simulink model "model_vec"  (R2022b)
settings: Solver=ode4  StartTime=0.0  StopTime=1.3  FixedStep=10e-6  RelTol=1e-3
InitFcn:
  | model_
values from neighbouring files (symbols this model uses):
  f = 50    [model_.m]
  i1dn = psi2n/Lm    [model_.m]
  i1qn = sqrt(Inmax^2-i1dn^2)    [model_.m]
  J = 0.4    [model_.m]
  L1 = L1sigma+Lm    (= 0.08477)    [model_.m]
  L1sigma = 2.27e-3    (= 0.00227)    [model_.m]
  L2 = L2sigma+Lm    (= 0.08477)    [model_.m]
  L2sigma = 2.27e-3    (= 0.00227)    [model_.m]
  Lm = 82.5e-3    (= 0.0825)    [model_.m]
  pp = 2    [model_.m]
  psi2n = sqrt(psi2nre^2+psi2nim^2)    [model_.m]
  R1 = 370e-3    (= 0.37)    [model_.m]
  R2 = 225e-3    (= 0.225)    [model_.m]
  R2_vec_model = 225e-3    (= 0.225)    [model_.m]
  sigma = 1-Lm^(2)/(L1*L2)    (= 0.0528396032209)    [model_.m]
  svmFrequency = 10000    [model_.m]
  Us = 400    [model_.m]
libraries: eeTransforms x16, spsMeanLib x7, slpidlib x4, simulink x2, dspsigops x2
(part 1 of 3)
settings Model: Creator=petrzakopal  LastModifiedBy=petrzakopal

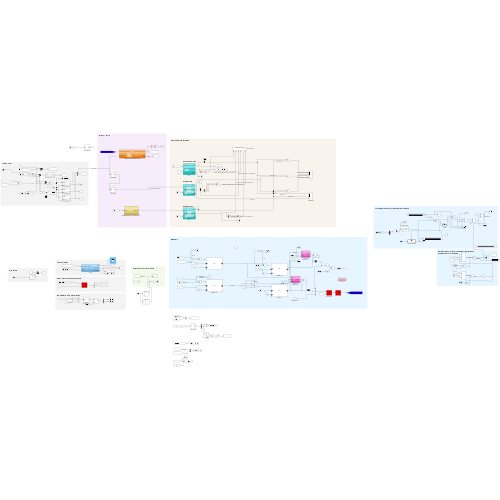
[thumbnail: Simulink's stored preview of the top-level diagram]
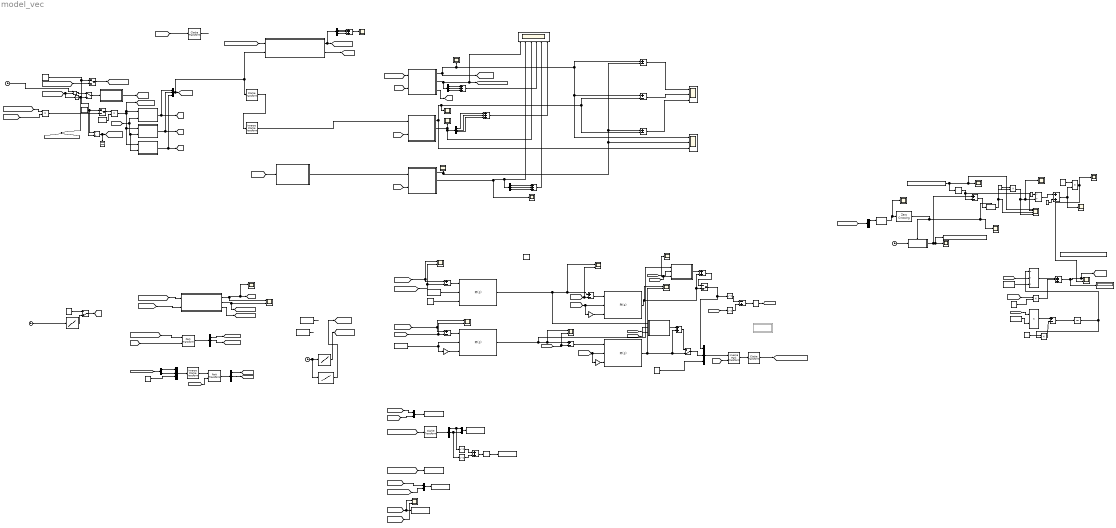
== system model_vec ==
  note: Voltage Source
  note: Goniometrický vstup
  note: Min-Max vstup
  note: Origin Voltage
  note: Regulators
  note: Regulators Control / Psi2, Omega
  note: I-n Motor Model
  note: Motor Stator Currents Transformation
  note: Motor Models and Validation
  note: Load Torque
  note: Invertor / Sources
  note: Moving frequency omega_s calculation for decoupling
  note: Psi2 alpha/beta to d/q transformation
  note: Moving frequency omega_s calculation for decoupling I-n model forward vector regulation
  1-D Lookup Table : Lookup_n-D  NumberOfTableDimensions=1  BreakpointsForDimension1=[0;1.02;1.020000000009;3]  Table=[0;0;40;40]  InternalRulePriority=Speed  RndMeth=Simplest
  1-D Lookup Table1 : Lookup_n-D  NumberOfTableDimensions=1  BreakpointsForDimension1=[0;0.45;0.4500001;1.5]  Table=[0;0;100;100]  InternalRulePriority=Speed  RndMeth=Simplest
  1-D Lookup Table2 : Lookup_n-D  NumberOfTableDimensions=1  BreakpointsForDimension1=[0;1.04;1.04000009;3]  Table=[0.9032;0.9032;0.6323;0.6323]  InternalRulePriority=Speed  RndMeth=Simplest
  ASM : Subsystem
  ASM1 : Subsystem
  ASM2 : Subsystem
  Add{,1..2,4,17} (5 alike) : Sum  Inputs=+++
  Add10 : Sum  Inputs=-+
  Add{8,11,14,16} (4 alike) : Sum
  Add{3,5..7,9,12..13,15,18} (9 alike) : Sum  Inputs=+-
  Checker Of Currents : Scope  NumInputPorts=6
  Clarke Transform{,1..3} (4 alike) : eeTransforms/Clarke Transform  PowerInvariant=off
      settings: LibrarySourceBlock=|
      | ee_sl_lib/Mathematical
      | Transforms/Clarke Transform
  Clock{,1..2,4} (4 alike) : Clock
  Constant : Constant
  Constant{1,3..4,6,25,32} (6 alike) : Constant  Value=0
  Constant10 : Constant  Value=(Lm*R2)/L2
  Constant11 : Constant  Value=R2/L2
  Constant15 : Constant  Value=sqrt(2)
  Constant16 : Constant  Value=50
  Constant17 : Constant  Value=220
  Constant18 : Constant  Value=1.5*i1dn
  Constant2 : Constant  Value=i1qn
  Constant20 : Constant  Value=psi2n
  Constant5 : Constant  Value=2
  Constant7 : Constant  Value=2*pi
  Constant8 : Constant  Value=(Lm*R2)/L2
  Constant9 : Constant  Value=pp
  Data Store Read : DataStoreRead  DataStoreName=reconstructed_voltage_zero_crossing_time  IndexOptions=Index vector (dialog)  Indices=1  OutputSizes=1
  Data Store Write : DataStoreWrite  DataStoreName=reconstructed_voltage_zero_crossing_time  IndexOptions=Index vector (dialog)  Indices=1  OutputSizes=1
  Data Store Memory : DataStoreMemory  DataStoreName=reconstructed_voltage_zero_crossing_time  WriteAfterWriteMsg=warning  ShowAdditionalParam=off
  Delay : Delay  DelayLength=15  InitialCondition=0
  Demux{,1..4,6..7,11} (8 alike) : Demux  Outputs=3
  Demux5 : Demux  Outputs=2
  Display : Display
  Display6 : Display
  Divide : Product  Inputs=*/
  Divide{1..2,4..6,12..13,15} (8 alike) : Product  Inputs=**
  Divide14 : Product  Inputs=*/
  Divide3 : Product  Inputs=/**
  For Transformations : Constant  Value=0
  Gain1 : Gain  Gain=-1
  Gain2 : Gain  Gain=-1
  Gain3 : Gain  Gain=-1
  Goniometric Space Vector Modulation Invertor : Subsystem
  I-n model : Subsystem
  Integrator : Integrator
  Integrator5 : Integrator  InitialCondition=20  UpperSaturationLimit=50  LowerSaturationLimit=-50
  Inverse Clarke Transform : eeTransforms/Inverse Clarke Transform  PowerInvariant=off
      settings: LibrarySourceBlock=|
      | ee_sl_lib/Mathematical
      | Transforms/Inverse
      | Clarke Transform
  Inverse Clarke Transform1 : eeTransforms/Inverse Clarke Transform  PowerInvariant=off
      settings: LibrarySourceBlock=|
      | ee_sl_lib/Mathematical
      | Transforms/Inverse
      | Clarke Transform
  Inverse Park Transform : eeTransforms/Inverse Park Transform  AxisAlignment=D-axis  PowerInvariant=off
      settings: LibrarySourceBlock=|
      | ee_sl_lib/Mathematical
      | Transforms/Inverse
      | Park Transform
  Inverse Park1 : Subsystem  Commented=on
  Manual Switch : ManualSwitch  CurrentSetting=0
  Manual Switch1 : ManualSwitch  CurrentSetting=0
  Manual Switch2 : ManualSwitch  CurrentSetting=0
  Manual Switch5 : ManualSwitch
  Manual Switch6 : ManualSwitch
  Manual Switch7 : ManualSwitch
  Math Function{,1,6..7} (4 alike) : Math  Operator=square
  Mean : spsMeanLib/Mean  Freq=50  Vinit=0  Ts=0
  Min-Max Method Space Vector Modulation Invertor : Subsystem
  Mux : Mux  Inputs=2
  Mux1 : Mux  Inputs=2
  Mux11 : Mux  Inputs=3
  Mux2 : Mux  Inputs=2
  Mux3 : Mux  Inputs=3
  Mux9 : Mux  Inputs=3
  Odvazbeni u1d (pricist k u1d) (minusy jsou uvnitr) : Subsystem
  Odvazbeni u1q (pricist k u1q) (minusy jsou uvnitr) : Subsystem
  Omega Checker : Scope  NumInputPorts=3
  Omega Subtract : Scope  NumInputPorts=3
  Omega*Time Calculation1 : Subsystem
  Park Transform : eeTransforms/Park Transform  AxisAlignment=D-axis  PowerInvariant=off
      settings: LibrarySourceBlock=|
      | ee_sl_lib/Mathematical
      | Transforms/Park Transform
  Park Transform1 : eeTransforms/Park Transform  AxisAlignment=Q-axis  PowerInvariant=off
      settings: LibrarySourceBlock=|
      | ee_sl_lib/Mathematical
      | Transforms/Park Transform
  Regulator Omega : slpidlib/PID Controller  Controller=PI  Form=Parallel  TimeDomain=Continuous-time  UseExternalTs=off  SampleTime=-1  IntegratorMethod=Forward Euler  FilterMethod=Forward Euler  ControllerParametersSource=internal  P=3.72e+3  I=4.65e6  UseKiTs=off  D=0  N=100  UseFilter=on  TunerSelectOption=Transfer Function Based (PID Tuner App)  InitialConditionSource=internal  InitialConditionForIntegrator=0  InitialConditionForFilter=0  DifferentiatorICPrevScaledInput=0  ExternalReset=none  TrackingMode=off  Kt=1  LimitOutput=on  SatLimitsSource=external  UpperSaturationLimit=inf  LowerSaturationLimit=-inf  LinearizeAsGain=on  AntiWindupMode=clamping  Kb=1  LimitIntegrator=off  UpperIntegratorSaturationLimit=inf  LowerIntegratorSaturationLimit=-inf  POutMin=[]  POutMax=[]  IOutMin=[]  IOutMax=[]  DOutMin=[]  DOutMax=[]  NOutMin=[]  NOutMax=[]  SumOutMin=[]  SumOutMax=[]  SaturationOutMin=[]  SaturationOutMax=[]  PParamMin=[]  PParamMax=[]  IParamMin=[]  IParamMax=[]  DParamMin=[]  DParamMax=[]  NParamMin=[]  NParamMax=[]  KbParamMin=[]  KbParamMax=[]  KtParamMin=[]  KtParamMax=[]  KbOutMin=[]  KbOutMax=[]  KtOutMin=[]  KtOutMax=[]  IntegratorOutMin=[]  IntegratorOutMax=[]  FilterOutMin=[]  FilterOutMax=[]  SumI1OutMin=[]  SumI1OutMax=[]  SumI2OutMin=[]  SumI2OutMax=[]  SumI3OutMin=[]  SumI3OutMax=[]  SumI4OutMin=[]  SumI4OutMax=[]  SumDOutMin=[]  SumDOutMax=[]  DifferentiatorOutMin=[]  DifferentiatorOutMax=[]  FilterDiffOutCoefMin=[]  FilterDiffOutCoefMax=[]  ReciprocalOutMin=[]  ReciprocalOutMax=[]  SumDenOutMin=[]  SumDenOutMax=[]  SumNumOutMin=[]  SumNumOutMax=[]  DivideOutMin=[]  DivideOutMax=[]  UdiffTsProdOutMin=[]  UdiffTsProdOutMax=[]  NTsProdOutMin=[]  NTsProdOutMax=[]  UintegralTsProdOutMin=[]  UintegralTsProdOutMax=[]  UngainTsProdOutMin=[]  UngainTsProdOutMax=[]  ClampingZeroOutDataTypeStr=Inherit: Inherit via back propagation  ClampingZeroOutMin=[]  ClampingZeroOutMax=[]  FilterDenConstantOutDataTypeStr=Inherit: Inherit via back propagation  FilterDenConstantOutMin=[]  FilterDenConstantOutMax=[]  PCopyOutDataTypeStr=Inherit: Inherit via back propagation  PCopyOutMin=[]  PCopyOutMax=[]  NCopyOutDataTypeStr=Inherit: Inherit via back propagation  NCopyOutMin=[]  NCopyOutMax=[]  IntegratorContinuousStateAttributes=''  IntegratorStateMustResolveToSignalObject=off  IntegratorRTWStateStorageClass=Auto  FilterContinuousStateAttributes=''  FilterStateMustResolveToSignalObject=off  FilterRTWStateStorageClass=Auto  ParallelPVariant=InternalParameters  IdealPVariant=Disabled  IVariant=InternalParameters  DVariant=Disabled  IntegratorVariant=Continuous  SatVariant=External  AWVariant=ContClampingParallel  PCopyVariant=Disabled  TRVariant=Disabled  FdbkBlocksVariant=Forward  IdealPFdbkVariant=Disabled  SatFdbkVariant=Disabled  DerivativeFilterVariant=Disabled  NVariant=Disabled  NCopyVariant=Disabled_SignalSpec  FilterICVariant=Disabled  IntegratorICVariant=InternalICs  ExternalResetVariant=Disabled  TRSumVariant=Passthrough  SumFdbkVariant=Disabled  SumVariant=Sum_PI  TsampFilterVariant=InternalTs  TsampNgainVariant=Passthrough  TsampIntegralVariant=Passthrough  ExternalSaturationOutDataTypeStr=Inherit: Same as second input
  Regulator Psi2 : slpidlib/PID Controller  Controller=PI  Form=Parallel  TimeDomain=Continuous-time  UseExternalTs=off  SampleTime=-1  IntegratorMethod=Forward Euler  FilterMethod=Forward Euler  ControllerParametersSource=internal  P=1.14e+4  I=3.03e4  UseKiTs=off  D=0  N=100  UseFilter=on  TunerSelectOption=Transfer Function Based (PID Tuner App)  InitialConditionSource=internal  InitialConditionForIntegrator=0  InitialConditionForFilter=0  DifferentiatorICPrevScaledInput=0  ExternalReset=none  TrackingMode=off  Kt=1  LimitOutput=on  SatLimitsSource=external  UpperSaturationLimit=inf  LowerSaturationLimit=-inf  LinearizeAsGain=on  AntiWindupMode=clamping  Kb=1  LimitIntegrator=off  UpperIntegratorSaturationLimit=inf  LowerIntegratorSaturationLimit=-inf  POutMin=[]  POutMax=[]  IOutMin=[]  IOutMax=[]  DOutMin=[]  DOutMax=[]  NOutMin=[]  NOutMax=[]  SumOutMin=[]  SumOutMax=[]  SaturationOutMin=[]  SaturationOutMax=[]  PParamMin=[]  PParamMax=[]  IParamMin=[]  IParamMax=[]  DParamMin=[]  DParamMax=[]  NParamMin=[]  NParamMax=[]  KbParamMin=[]  KbParamMax=[]  KtParamMin=[]  KtParamMax=[]  KbOutMin=[]  KbOutMax=[]  KtOutMin=[]  KtOutMax=[]  IntegratorOutMin=[]  IntegratorOutMax=[]  FilterOutMin=[]  FilterOutMax=[]  SumI1OutMin=[]  SumI1OutMax=[]  SumI2OutMin=[]  SumI2OutMax=[]  SumI3OutMin=[]  SumI3OutMax=[]  SumI4OutMin=[]  SumI4OutMax=[]  SumDOutMin=[]  SumDOutMax=[]  DifferentiatorOutMin=[]  DifferentiatorOutMax=[]  FilterDiffOutCoefMin=[]  FilterDiffOutCoefMax=[]  ReciprocalOutMin=[]  ReciprocalOutMax=[]  SumDenOutMin=[]  SumDenOutMax=[]  SumNumOutMin=[]  SumNumOutMax=[]  DivideOutMin=[]  DivideOutMax=[]  UdiffTsProdOutMin=[]  UdiffTsProdOutMax=[]  NTsProdOutMin=[]  NTsProdOutMax=[]  UintegralTsProdOutMin=[]  UintegralTsProdOutMax=[]  UngainTsProdOutMin=[]  UngainTsProdOutMax=[]  ClampingZeroOutDataTypeStr=Inherit: Inherit via back propagation  ClampingZeroOutMin=[]  ClampingZeroOutMax=[]  FilterDenConstantOutDataTypeStr=Inherit: Inherit via back propagation  FilterDenConstantOutMin=[]  FilterDenConstantOutMax=[]  PCopyOutDataTypeStr=Inherit: Inherit via back propagation  PCopyOutMin=[]  PCopyOutMax=[]  NCopyOutDataTypeStr=Inherit: Inherit via back propagation  NCopyOutMin=[]  NCopyOutMax=[]  IntegratorContinuousStateAttributes=''  IntegratorStateMustResolveToSignalObject=off  IntegratorRTWStateStorageClass=Auto  FilterContinuousStateAttributes=''  FilterStateMustResolveToSignalObject=off  FilterRTWStateStorageClass=Auto  ParallelPVariant=InternalParameters  IdealPVariant=Disabled  IVariant=InternalParameters  DVariant=Disabled  IntegratorVariant=Continuous  SatVariant=External  AWVariant=ContClampingParallel  PCopyVariant=Disabled  TRVariant=Disabled  FdbkBlocksVariant=Forward  IdealPFdbkVariant=Disabled  SatFdbkVariant=Disabled  DerivativeFilterVariant=Disabled  NVariant=Disabled  NCopyVariant=Disabled_SignalSpec  FilterICVariant=Disabled  IntegratorICVariant=InternalICs  ExternalResetVariant=Disabled  TRSumVariant=Passthrough  SumFdbkVariant=Disabled  SumVariant=Sum_PI  TsampFilterVariant=InternalTs  TsampNgainVariant=Passthrough  TsampIntegralVariant=Passthrough  ExternalSaturationOutDataTypeStr=Inherit: Same as second input
  Regulator i1d : slpidlib/PID Controller  Controller=PI  Form=Parallel  TimeDomain=Continuous-time  UseExternalTs=off  SampleTime=-1  IntegratorMethod=Forward Euler  FilterMethod=Forward Euler  ControllerParametersSource=internal  P=22.39  I=2.91e+3  UseKiTs=off  D=0  N=100  UseFilter=on  TunerSelectOption=Transfer Function Based (PID Tuner App)  InitialConditionSource=internal  InitialConditionForIntegrator=0  InitialConditionForFilter=0  DifferentiatorICPrevScaledInput=0  ExternalReset=none  TrackingMode=off  Kt=1  LimitOutput=on  SatLimitsSource=external  UpperSaturationLimit=inf  LowerSaturationLimit=-inf  LinearizeAsGain=on  AntiWindupMode=clamping  Kb=1  LimitIntegrator=off  UpperIntegratorSaturationLimit=inf  LowerIntegratorSaturationLimit=-inf  POutMin=[]  POutMax=[]  IOutMin=[]  IOutMax=[]  DOutMin=[]  DOutMax=[]  NOutMin=[]  NOutMax=[]  SumOutMin=[]  SumOutMax=[]  SaturationOutMin=[]  SaturationOutMax=[]  PParamMin=[]  PParamMax=[]  IParamMin=[]  IParamMax=[]  DParamMin=[]  DParamMax=[]  NParamMin=[]  NParamMax=[]  KbParamMin=[]  KbParamMax=[]  KtParamMin=[]  KtParamMax=[]  KbOutMin=[]  KbOutMax=[]  KtOutMin=[]  KtOutMax=[]  IntegratorOutMin=[]  IntegratorOutMax=[]  FilterOutMin=[]  FilterOutMax=[]  SumI1OutMin=[]  SumI1OutMax=[]  SumI2OutMin=[]  SumI2OutMax=[]  SumI3OutMin=[]  SumI3OutMax=[]  SumI4OutMin=[]  SumI4OutMax=[]  SumDOutMin=[]  SumDOutMax=[]  DifferentiatorOutMin=[]  DifferentiatorOutMax=[]  FilterDiffOutCoefMin=[]  FilterDiffOutCoefMax=[]  ReciprocalOutMin=[]  ReciprocalOutMax=[]  SumDenOutMin=[]  SumDenOutMax=[]  SumNumOutMin=[]  SumNumOutMax=[]  DivideOutMin=[]  DivideOutMax=[]  UdiffTsProdOutMin=[]  UdiffTsProdOutMax=[]  NTsProdOutMin=[]  NTsProdOutMax=[]  UintegralTsProdOutMin=[]  UintegralTsProdOutMax=[]  UngainTsProdOutMin=[]  UngainTsProdOutMax=[]  ClampingZeroOutDataTypeStr=Inherit: Inherit via back propagation  ClampingZeroOutMin=[]  ClampingZeroOutMax=[]  FilterDenConstantOutDataTypeStr=Inherit: Inherit via back propagation  FilterDenConstantOutMin=[]  FilterDenConstantOutMax=[]  PCopyOutDataTypeStr=Inherit: Inherit via back propagation  PCopyOutMin=[]  PCopyOutMax=[]  NCopyOutDataTypeStr=Inherit: Inherit via back propagation  NCopyOutMin=[]  NCopyOutMax=[]  IntegratorContinuousStateAttributes=''  IntegratorStateMustResolveToSignalObject=off  IntegratorRTWStateStorageClass=Auto  FilterContinuousStateAttributes=''  FilterStateMustResolveToSignalObject=off  FilterRTWStateStorageClass=Auto  ParallelPVariant=InternalParameters  IdealPVariant=Disabled  IVariant=InternalParameters  DVariant=Disabled  IntegratorVariant=Continuous  SatVariant=External  AWVariant=ContClampingParallel  PCopyVariant=Disabled  TRVariant=Disabled  FdbkBlocksVariant=Forward  IdealPFdbkVariant=Disabled  SatFdbkVariant=Disabled  DerivativeFilterVariant=Disabled  NVariant=Disabled  NCopyVariant=Disabled_SignalSpec  FilterICVariant=Disabled  IntegratorICVariant=InternalICs  ExternalResetVariant=Disabled  TRSumVariant=Passthrough  SumFdbkVariant=Disabled  SumVariant=Sum_PI  TsampFilterVariant=InternalTs  TsampNgainVariant=Passthrough  TsampIntegralVariant=Passthrough  ExternalSaturationOutDataTypeStr=Inherit: Same as second input
  Regulator i1q : slpidlib/PID Controller  Controller=PI  Form=Parallel  TimeDomain=Continuous-time  UseExternalTs=off  SampleTime=-1  IntegratorMethod=Forward Euler  FilterMethod=Forward Euler  ControllerParametersSource=internal  P=22.39  I=2.91e+3  UseKiTs=off  D=0  N=100  UseFilter=on  TunerSelectOption=Transfer Function Based (PID Tuner App)  InitialConditionSource=internal  InitialConditionForIntegrator=0  InitialConditionForFilter=0  DifferentiatorICPrevScaledInput=0  ExternalReset=none  TrackingMode=off  Kt=1  LimitOutput=on  SatLimitsSource=external  UpperSaturationLimit=inf  LowerSaturationLimit=-inf  LinearizeAsGain=on  AntiWindupMode=clamping  Kb=1  LimitIntegrator=off  UpperIntegratorSaturationLimit=inf  LowerIntegratorSaturationLimit=-inf  POutMin=[]  POutMax=[]  IOutMin=[]  IOutMax=[]  DOutMin=[]  DOutMax=[]  NOutMin=[]  NOutMax=[]  SumOutMin=[]  SumOutMax=[]  SaturationOutMin=[]  SaturationOutMax=[]  PParamMin=[]  PParamMax=[]  IParamMin=[]  IParamMax=[]  DParamMin=[]  DParamMax=[]  NParamMin=[]  NParamMax=[]  KbParamMin=[]  KbParamMax=[]  KtParamMin=[]  KtParamMax=[]  KbOutMin=[]  KbOutMax=[]  KtOutMin=[]  KtOutMax=[]  IntegratorOutMin=[]  IntegratorOutMax=[]  FilterOutMin=[]  FilterOutMax=[]  SumI1OutMin=[]  SumI1OutMax=[]  SumI2OutMin=[]  SumI2OutMax=[]  SumI3OutMin=[]  SumI3OutMax=[]  SumI4OutMin=[]  SumI4OutMax=[]  SumDOutMin=[]  SumDOutMax=[]  DifferentiatorOutMin=[]  DifferentiatorOutMax=[]  FilterDiffOutCoefMin=[]  FilterDiffOutCoefMax=[]  ReciprocalOutMin=[]  ReciprocalOutMax=[]  SumDenOutMin=[]  SumDenOutMax=[]  SumNumOutMin=[]  SumNumOutMax=[]  DivideOutMin=[]  DivideOutMax=[]  UdiffTsProdOutMin=[]  UdiffTsProdOutMax=[]  NTsProdOutMin=[]  NTsProdOutMax=[]  UintegralTsProdOutMin=[]  UintegralTsProdOutMax=[]  UngainTsProdOutMin=[]  UngainTsProdOutMax=[]  ClampingZeroOutDataTypeStr=Inherit: Inherit via back propagation  ClampingZeroOutMin=[]  ClampingZeroOutMax=[]  FilterDenConstantOutDataTypeStr=Inherit: Inherit via back propagation  FilterDenConstantOutMin=[]  FilterDenConstantOutMax=[]  PCopyOutDataTypeStr=Inherit: Inherit via back propagation  PCopyOutMin=[]  PCopyOutMax=[]  NCopyOutDataTypeStr=Inherit: Inherit via back propagation  NCopyOutMin=[]  NCopyOutMax=[]  IntegratorContinuousStateAttributes=''  IntegratorStateMustResolveToSignalObject=off  IntegratorRTWStateStorageClass=Auto  FilterContinuousStateAttributes=''  FilterStateMustResolveToSignalObject=off  FilterRTWStateStorageClass=Auto  ParallelPVariant=InternalParameters  IdealPVariant=Disabled  IVariant=InternalParameters  DVariant=Disabled  IntegratorVariant=Continuous  SatVariant=External  AWVariant=ContClampingParallel  PCopyVariant=Disabled  TRVariant=Disabled  FdbkBlocksVariant=Forward  IdealPFdbkVariant=Disabled  SatFdbkVariant=Disabled  DerivativeFilterVariant=Disabled  NVariant=Disabled  NCopyVariant=Disabled_SignalSpec  FilterICVariant=Disabled  IntegratorICVariant=InternalICs  ExternalResetVariant=Disabled  TRSumVariant=Passthrough  SumFdbkVariant=Disabled  SumVariant=Sum_PI  TsampFilterVariant=InternalTs  TsampNgainVariant=Passthrough  TsampIntegralVariant=Passthrough  ExternalSaturationOutDataTypeStr=Inherit: Same as second input
  Sample and Hold : dspsigops/Sample and Hold  trig=Rising edge  initCond=999999999  latchinput=off
  Scope{1..3,5..10,12..15,23} (14 alike) : Scope
  Scope11 : Scope  NumInputPorts=4
  Scope{4,16..17,24,26..30} (9 alike) : Scope  NumInputPorts=2
  Sqrt : Sqrt
  Sqrt1 : Sqrt
  To Workspace : ToWorkspace  VariableName=omega_wanted_real  SaveFormat=Timeseries  SampleTime=-1
  To Workspace1 : ToWorkspace  VariableName=i_1alpha_1beta  SaveFormat=Timeseries  SampleTime=-1
  To Workspace2 : ToWorkspace  VariableName=i_1_module  SaveFormat=Timeseries  SampleTime=-1
  To Workspace3 : ToWorkspace  VariableName=Psi_2_alpha_beta  SaveFormat=Timeseries  SampleTime=-1
  To Workspace4 : ToWorkspace  VariableName=Psi_2_wanted_real  SaveFormat=Timeseries  SampleTime=-1
  To Workspace5 : ToWorkspace  VariableName=Mh  SaveFormat=Timeseries  SampleTime=-1
  Triggered Subsystem : Subsystem  TreatAsAtomicUnit=on
  Zero Crossing : dspsigops/Zero Crossing  InputProcessing=Columns as channels (frame based)
  u4 : Subsystem
  u5 : Subsystem
  u6 : Subsystem
  wires:
  ASM/1(Omega) -> [Omega_real], Omega Checker/1, Add12/1, Add7/1, Scope23/1  "Omega_gonio"
  ASM/2("Measured Motor Current Ia, Ib, Ic") -> Demux2/1, Checker Of Currents/1, [measured_motor_current]  "Measured Motor Current I1a, I1b, I1c Gonio Invertor"
  [u_reconstruction] -> ASM/1("Voltage Input Ua, Ub, Uc")
  u6/1(u3) -> Mux9/3, [u3]
  Divide13/1 -> Manual Switch7/1
  Mux9/1 -> Goniometric Space Vector Modulation Invertor/2(Test Ua Ub Uc), Clarke Transform2/1, [u_1source]  "u_1source_origin"
  Constant16/1 -> Manual Switch6/1, Divide14/2
  [omega_t] -> u4/2(omega_t), u6/2(omega_t), u5/2(omega_t)
  [input_variable_frequency] -> Manual Switch6/2
  Integrator5/1 -> [input_variable_frequency_after_int], Manual Switch7/2
  Divide14/1 -> Display6/1, [U_f_nominal]
  Divide12/1 -> [input_U_amplitude], u4/1(amplitude), u6/1(amplitude), u5/1(amplitude)
  Clock4/1 -> Divide13/1
  Omega*Time Calculation1/1(omega_t) -> [omega_t]
  u4/1(u1) -> Mux9/1, [u1]
  Constant15/1 -> Divide12/2
  Divide15/1 -> Manual Switch5/2  "U"
  Manual Switch7/1 -> Omega*Time Calculation1/1(frequency)
  Constant17/1 -> Manual Switch5/1, Divide14/1
  [input_variable_frequency] -> Divide15/1
  Manual Switch5/1 -> Divide12/1
  u5/1(u2) -> [u2], Mux9/2
  Manual Switch6/1 -> [input_frequency]
  [U_f_nominal] -> Divide15/2
  [input_frequency] -> Divide13/2, Integrator5/1
  Goniometric Space Vector Modulation Invertor/1("Invertor Voltage Output Ua, Ub, Uc") -> Demux/1, [u_reconstruction]  "Invertor Voltage Output Ua, Ub, Uc Goniometric"
  [u_1source] -> Clarke Transform/1
  [measured_motor_current] -> I-n model/1("Measured Motor Current Ia, Ib, Ic")
  I-n model/1(Theta) -> Scope24/1, Scope17/1, [Theta]
  [Omega_real] -> I-n model/2(Omega)
  I-n model/2(Psi_2_module) -> [Psi_2_module_real], Scope24/2  "Psi_2_module_real"
  [measured_motor_current] -> Park Transform/1
  [Theta] -> Park Transform/2
  Park Transform/1 -> Demux11/1
  Goniometric Space Vector Modulation Invertor/2(uDCmax) -> [uDCmax]  "uDCmax"
  Demux11/1 -> [i1d_real]
  Demux11/2 -> [i1q_real]
  [Theta] -> Inverse Park Transform/2
  Regulator i1d/1 -> Manual Switch1/2, Add11/2, Scope28/1  "u1d"
  Add9/1 -> Regulator i1d/1
  Regulator Psi2/1 -> Odvazbeni u1q (pricist k u1q) (minusy jsou uvnitr)/1(i1d), Scope26/1, Add9/1  "i1d_wanted"
  [i1d_real] -> Scope26/2, Add9/2  "i1d_real"
  [uDCmax] -> Gain1/1, Regulator i1d/2
  [uDCmax] -> Math Function6/1
  Math Function6/1 -> Add10/2
  Math Function7/1 -> Add10/1
  Mux11/1 -> Inverse Park Transform/1
  Add10/1 -> Sqrt1/1
  Sqrt1/1 -> [u1q_max]
  Constant32/1 -> Regulator Psi2/3
  [psi2_wanted] -> Scope29/1, Add5/1  "Psi2_wanted"
  [u1q_max] -> Gain3/1, Regulator i1q/2
  Gain3/1 -> Regulator i1q/3
  [i1q_real] -> Scope27/2, Add3/2  "i1q_real"
  Constant18/1 -> Regulator Psi2/2
  Constant2/1 -> Regulator Omega/2, Gain2/1
  Gain2/1 -> Regulator Omega/3
  [Omega_wanted] -> Add6/1, Scope30/1  "Omega_wanted"
  Regulator i1q/1 -> Manual Switch2/2, Add14/2, Scope28/2  "u1q"
  For Transformations/1 -> Mux11/3
  [Psi_2_module_real] -> Scope29/2, Add5/2  "Psi2_real"
  Add5/1 -> Regulator Psi2/1
  Add6/1 -> Regulator Omega/1
  [Omega_real] -> Scope30/2, Add6/2  "Omega_real"
  Inverse Park Transform/1 -> Clarke Transform1/1
  Clarke Transform1/1 -> [u1_alpha_beta_0_to_inverter]
  Add3/1 -> Regulator i1q/1  "u1q"
  Clarke Transform/1 -> ?
  Demux/1 -> Add/1
  Demux/2 -> Add/2
  Demux/3 -> Add/3
  Add/1 -> Scope2/1  "Invertor Voltage Output Ua, Ub, Uc Addition"
  [u1_alpha_beta_0_to_inverter] -> Goniometric Space Vector Modulation Invertor/1("Invertor Voltage Input Ualpha, Ubeta")
  [u_1source] -> Min-Max Method Space Vector Modulation Invertor/1(Ua Ub Uc)
  Min-Max Method Space Vector Modulation Invertor/1(u_reconstruction) -> ASM1/1("Voltage Input Ua, Ub, Uc")
  ASM1/1(Omega) -> Add7/2, Add13/1, Omega Checker/2, Scope1/1  "Omega_min_max"
  ASM1/2("Measured Motor Current Ia, Ib, Ic") -> Scope3/1, Checker Of Currents/2, Demux1/1  "Measured Motor Current I1a, I1b, I1c Min Max Invertor"
  Add1/1 -> Checker Of Currents/5  "Addition of Motor Measured Currents I1a, I1b, I1c Min Max Invertor"
  Demux1/1 -> Add1/1
  Demux1/2 -> Add1/2
  Demux1/3 -> Add1/3
  Demux2/1 -> Add2/1
  Demux2/2 -> Add2/2
  Demux2/3 -> Add2/3
  Add2/1 -> Checker Of Currents/4  "Addition of Motor Measured Currents I1a, I1b, I1c Gonio Invertor"
  ASM2/2("Measured Motor Current Ia, Ib, Ic") -> Checker Of Currents/3, Demux3/1, Scope5/1  "Measured Motor Current I1a, I1b, I1c Origin Voltage"
  Demux3/1 -> Add4/1
  Demux3/2 -> Add4/2
  Demux3/3 -> Add4/3
  Add4/1 -> Checker Of Currents/6  "Addition of Motor Measured Currents I1a, I1b, I1c Origin Voltage"
  ASM2/1(Omega) -> Omega Checker/3, Add12/2, Add13/2, Scope7/1  "Omega_origin"
  Add7/1 -> Omega Subtract/1  "Omega gonio minus Omega Min Max"
  Add12/1 -> Omega Subtract/2  "Omega gonio minus Omega Origin"
  Add13/1 -> Omega Subtract/3  "Omega Min Max minus Omega Origin"
  Clarke Transform2/1 -> Inverse Clarke Transform/1
  Inverse Clarke Transform/1 -> ASM2/1("Voltage Input Ua, Ub, Uc")  "u_1source after transformation"
  Constant20/1 -> ?  "Psi2_wanted"
  Constant25/1 -> ?  "Omega_wanted"
  [Omega_wanted] -> Mux/1  "Omega_wanted"
  [Omega_real] -> Mux/2  "Omega_real"
  Mux/1 -> To Workspace/1
  [measured_motor_current] -> Clarke Transform3/1
  Clarke Transform3/1 -> Demux4/1
  Demux4/1 -> Math Function/1, Mux1/1
  Demux4/2 -> Math Function1/1, Mux1/2
  Mux1/1 -> To Workspace1/1
  Math Function/1 -> Add8/1
  Math Function1/1 -> Add8/2
  Add8/1 -> Sqrt/1
  Sqrt/1 -> To Workspace2/1
  I-n model/3(Psi_2_alpha_beta) -> [Psi_2_alpha_beta]
  [Psi_2_alpha_beta] -> To Workspace3/1
  [psi2_wanted] -> Mux2/1  "Psi2_wanted"
  [Psi_2_module_real] -> Mux2/2  "Psi2_real"
  Mux2/1 -> To Workspace4/1
  Manual Switch/1 -> [Mz]
  1-D Lookup Table/1 -> Manual Switch/2
  Clock/1 -> 1-D Lookup Table/1
  Constant4/1 -> Manual Switch/1
  [Mz] -> ASM/2(Mz)
  [Mz] -> ASM2/2(Mz)
  [Mz] -> ASM1/2(Mz)
  ASM/3(Mhnaci) -> [Mh]
  [Mh] -> Scope4/1, To Workspace5/1  "Mh"
  [Psi_2_alpha_beta] -> Demux5/1
  Demux5/1 -> Mux3/1
  Demux5/2 -> Mux3/2
  Constant3/1 -> Mux3/3  "i1q_wanted"
  Mux3/1 -> Inverse Clarke Transform1/1
  Inverse Clarke Transform1/1 -> Park Transform1/1
  [Theta] -> Park Transform1/2
  Park Transform1/1 -> Demux6/1
  Demux6/1 -> [Psi2_d]
  Demux6/2 -> [Psi2_q]
  [Psi2_d] -> Odvazbeni u1d (pricist k u1d) (minusy jsou uvnitr)/2(psi2d)
  Odvazbeni u1d (pricist k u1d) (minusy jsou uvnitr)/1(odvazbeni) -> Add11/1
  [Psi2_d] -> Odvazbeni u1q (pricist k u1q) (minusy jsou uvnitr)/2(psi2d)
  Odvazbeni u1q (pricist k u1q) (minusy jsou uvnitr)/1(odvazbeni) -> Add14/1
  Clock1/1 -> 1-D Lookup Table2/1, 1-D Lookup Table1/1
  1-D Lookup Table1/1 -> [Omega_wanted]
  Regulator Omega/1 -> Odvazbeni u1d (pricist k u1d) (minusy jsou uvnitr)/1(i1q), Add3/1, Scope27/1  "i1q_wanted"
  Gain1/1 -> Regulator i1d/3
  [u_reconstruction] -> Demux7/1
  Demux7/1 -> Mean/1
  Clock2/1 -> Triggered Subsystem/1(In1)
  Mean/1 -> Scope8/1, Zero Crossing/1  "ua_reconstructed_mean"
  Triggered Subsystem/1(Out1) -> Add15/1, Data Store Write/1, Scope6/1
  Data Store Read/1 -> Scope11/1, Scope9/1, Delay/1
  Sample and Hold/1 -> Divide1/2, Scope11/3
  Constant/1 -> Divide/1
  Constant5/1 -> Divide1/1
  Delay/1 -> Scope11/2, Add15/2
  Zero Crossing/1 -> Scope12/1, Sample and Hold/Trigger, Triggered Subsystem/Trigger
  Divide1/1 -> Scope11/4, Scope14/1, Divide/2
  Add15/1 -> Sample and Hold/1
  Add16/1 -> Divide2/2, Scope13/1
  [omega_s] -> Scope10/1, Odvazbeni u1d (pricist k u1d) (minusy jsou uvnitr)/3(omega_s)
  [omega_s] -> Odvazbeni u1q (pricist k u1q) (minusy jsou uvnitr)/3(omega_s)
  Add14/1 -> Manual Switch2/1
  Divide/1 -> Add16/1
  Constant6/1 -> Add16/2
  1-D Lookup Table2/1 -> [psi2_wanted]
  [Mz] -> Scope4/2  "Mz"
  Add11/1 -> Manual Switch1/1  "u1d"
  Manual Switch1/1 -> Mux11/1, Math Function7/1
  Manual Switch2/1 -> Mux11/2
  Constant7/1 -> Divide2/1
  Divide2/1 -> Scope16/2, Scope15/1  "omega_s (z prubehu napeti)"
  [i1q_real] -> Divide3/2  "i1q_real"
  Constant8/1 -> Divide3/3
  Divide3/1 -> Add17/1  "omega_slip"
  [Omega_real] -> Divide4/1  "Omega_real"
  Constant9/1 -> Divide4/2
  Divide4/1 -> Add17/2
  Add17/1 -> Display/1, [omega_s], Scope16/1  "omega_s (odhadnuta)"
  [i1d_real] -> Divide5/1  "i1q_real"
  Constant10/1 -> Divide5/2
  Divide5/1 -> Add18/1  "omega_slip"
  Constant11/1 -> Divide6/1
  Divide6/1 -> Add18/2
  Add18/1 -> Integrator/1  "dPsi_2_d"
  Integrator/1 -> Divide6/2, Divide3/1

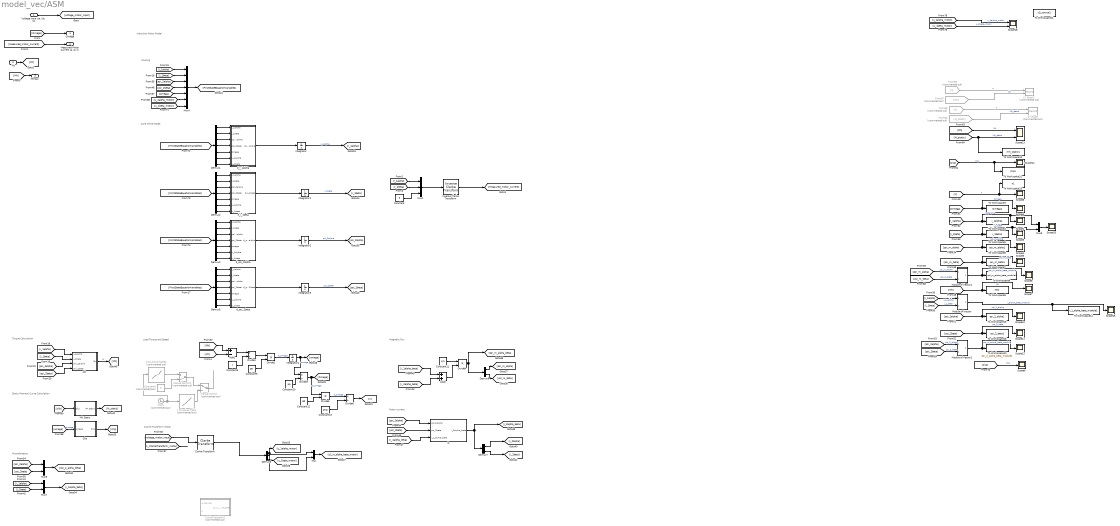
== system model_vec/ASM ==
  note: Clarke Transform Motor
  note: Induction Motor Model
  note: Rotor current
  note: Magnetic flux
  note: Static Moment Curve Calculation
  note: Routing
  note: Miscellaneous
  note: Load Torque and Speed
  note: Torque Calculation
  note: Core of the Model
  "Voltage Input Ua, Ub, Uc" : Inport
  Mz : Inport  Port=2
  1-D Lookup Table : Lookup_n-D  Commented=on  NumberOfTableDimensions=1  BreakpointsForDimension1=[0;1.00001;1.001;10]  Table=[0;0;25;25]  InternalRulePriority=Speed  RndMeth=Simplest
  1-D Lookup Table2 : Lookup_n-D  Commented=on  NumberOfTableDimensions=1  BreakpointsForDimension1=[1;2;10]  Table=[0;0;78.48]  InternalRulePriority=Speed  RndMeth=Simplest
  Add1 : Sum  Inputs=+-
  Add2 : Sum
  Clarke Transform : eeTransforms/Clarke Transform  PowerInvariant=off
      settings: LibrarySourceBlock=|
      | ee_sl_lib/Mathematical
      | Transforms/Clarke Transform
  ClarkeTransform1 : Subsystem  Commented=on
  Clock : Clock  Commented=on
  Constant : Constant  Value=0
  Constant10 : Constant  Value=pp
  Constant11 : Constant  Value=Lm
  Constant12 : Constant  Value=60
  Constant13 : Constant  Value=2*pi
  Constant4 : Constant  Commented=on  Value=0
  Constant5 : Constant  Value=J
  Constant6 : Constant  Value=pp
  Demux{1..3,5} (4 alike) : Demux  Outputs=7
  Demux6 : Demux  Outputs=3
  Demux7 : Demux  Outputs=2
  Demux8 : Demux  Outputs=2
  Divide1 : Product  Inputs=*/
  Divide2 : Product  Inputs=**
  Divide3 : Product  Inputs=*/
  Divide4 : Product  Inputs=**
  Divide5 : Product  Inputs=**
  Divide6 : Product  Inputs=*/
  From62 : From  Commented=on  GotoTag=M_static
  From65 : From  Commented=on  GotoTag=n
  From67 : From  Commented=on  GotoTag=Mh
  From69 : From  Commented=on  GotoTag=n
  Integrator{,1..4} (5 alike) : Integrator
  Inverse Clarke Transform : eeTransforms/Inverse Clarke Transform  PowerInvariant=off
      settings: LibrarySourceBlock=|
      | ee_sl_lib/Mathematical
      | Transforms/Inverse
      | Clarke Transform
  Manual Switch : ManualSwitch  Commented=on
  Manual Switch1 : ManualSwitch  Commented=on  CurrentSetting=0
  Mh : Subsystem
  Mh Static : Subsystem
  Module of Vector : Subsystem
  Module of Vector1 : Subsystem
  Module of Vector2 : Subsystem
  Mux{,6..8} (4 alike) : Mux  Inputs=2
  Mux1 : Mux  Inputs=3
  Mux4 : Mux  Inputs=7
  Scope{1..12,14..15,20} (15 alike) : Scope
  Scope13 : Scope  NumInputPorts=2
  Scope18 : Scope  NumInputPorts=2
  Slip : Subsystem
  To Workspace10 : ToWorkspace  VariableName=psi_2_alpha_beta_module1  SaveFormat=Timeseries  SampleTime=-1
  To Workspace11 : ToWorkspace  VariableName=slip1  SaveFormat=Timeseries  SampleTime=-1
  To Workspace12 : ToWorkspace  VariableName=mh_static1  SaveFormat=Timeseries  SampleTime=-1
  To Workspace13 : ToWorkspace  VariableName=n1  SaveFormat=Timeseries  SampleTime=-1
  To Workspace14 : ToWorkspace  VariableName=i_1_alpha_beta_module1  SaveFormat=Timeseries  SampleTime=-1
  To Workspace15 : ToWorkspace  VariableName=psi_2_alpha1  SaveFormat=Timeseries  SampleTime=-1
  To Workspace16 : ToWorkspace  VariableName=psi_2_beta1  SaveFormat=Timeseries  SampleTime=-1
  To Workspace21 : ToWorkspace  VariableName=u3_source1  SaveFormat=Timeseries  SampleTime=-1
  To Workspace3 : ToWorkspace  VariableName=Omega1  SaveFormat=Timeseries  SampleTime=-1
  To Workspace4 : ToWorkspace  VariableName=i_1alpha1  SaveFormat=Timeseries  SampleTime=-1
  To Workspace5 : ToWorkspace  VariableName=i_1beta1  SaveFormat=Timeseries  SampleTime=-1
  To Workspace6 : ToWorkspace  VariableName=psi_m_alpha1  SaveFormat=Timeseries  SampleTime=-1
  To Workspace7 : ToWorkspace  VariableName=psi_m_beta1  SaveFormat=Timeseries  SampleTime=-1
  To Workspace8 : ToWorkspace  VariableName=psi_m_alpha_beta_module1  SaveFormat=Timeseries  SampleTime=-1
  To Workspace9 : ToWorkspace  VariableName=Mh1  SaveFormat=Timeseries  SampleTime=-1
  XY Graph : Record  Commented=on  FileSettingsInternal="{\"entries\":[{\"content\":{\"excelSettings\":{\"content\":{},\"type\":\"Streamout.ExcelSettings\"}},\"type\":\"Streamout.FileSettingStorage\",\"uuid\":\"c8a957cb-e6b8-4b51-a749-9efeca271d01\"}],\"packageUris\":[\"http://schema.mathworks.com/mf0/streamout_blocks/R2020a\"],\"version\":\"1.0\"}"  Layout=[1 1]  SignalsInternal="{\"entries\":[{\"content\":{\"signals\":[{\"content\":{\"blockPath\":[\"model_vec/ASM/XY Graph\"],\"channel\":[],\"dimensions\":[1],\"domain\":\"model_vec/ASM/XY Graph\",\"lineColor\":\"#a2142f\",\"plots\":[1],\"port\":1,\"sid\":[],\"signalID\":890,\"signalName\":\"n\"},\"type\":\"RecordBlkView.Signal\",\"uuid\":\"11359bd5-c93e-4a74-89aa-0be98840e253\"},{\"content\":{\"blockPath\":[\"model_vec/ASM/XY Graph\"],\"channel\":[],\"dimensions\":[1],\"domain\":\"model_vec/ASM/XY Graph\",\"lineColor\":\"#139fff\",\"plots\":[1],\"port\":2,\"sid\":[],\"signalID\":893,\"signalName\":\"Mh_static\"},\"type\":\"RecordBlkView.Signal\",\"uuid\":\"04c46477-7421-4e27-bac9-c5ac67648501\"}]},\"type\":\"RecordBlkView.InputSignals\",\"uuid\":\"446bd9f3-5f9d-4bbf-bb20-50a1a8788ada\"}],\"packageUris\":[\"http://schema.mathworks.com/mf0/streamout_blocks/R2020a\"],\"version\":\"1.0\"}"  VisualizationBindings="{\"xyplotplugin\":{\"info\":[{\"series\":[{\"bindingParametersList\":[{\"parameter\":\"X-Axis\",\"signalID\":890,\"signalName\":\"n\"},{\"parameter\":\"Y-Axis\",\"signalID\":893,\"signalName\":\"Mh_static\"}],\"seriesID\":16905}],\"subplotID\":1}]}}"  CompatibilityTag=XY
  XY Graph1 : Record  Commented=on  FileSettingsInternal="{\"entries\":[{\"content\":{\"excelSettings\":{\"content\":{},\"type\":\"Streamout.ExcelSettings\"}},\"type\":\"Streamout.FileSettingStorage\",\"uuid\":\"ece9c392-97d7-42b2-8769-a4c18fe8b02c\"}],\"packageUris\":[\"http://schema.mathworks.com/mf0/streamout_blocks/R2020a\"],\"version\":\"1.0\"}"  Layout=[1 1]  SignalsInternal="{\"entries\":[{\"content\":{\"signals\":[{\"content\":{\"blockPath\":[\"model_vec/ASM/XY Graph1\"],\"channel\":[],\"dimensions\":[1],\"domain\":\"model_vec/ASM/XY Graph1\",\"lineColor\":\"#a2142f\",\"plots\":[1],\"port\":1,\"sid\":[],\"signalID\":898,\"signalName\":\"n\"},\"type\":\"RecordBlkView.Signal\",\"uuid\":\"95364762-3763-4469-81c3-67c64f8346b3\"},{\"content\":{\"blockPath\":[\"model_vec/ASM/XY Graph1\"],\"channel\":[],\"dimensions\":[1],\"domain\":\"model_vec/ASM/XY Graph1\",\"lineColor\":\"#139fff\",\"plots\":[1],\"port\":2,\"sid\":[],\"signalID\":901,\"signalName\":\"Mh\"},\"type\":\"RecordBlkView.Signal\",\"uuid\":\"1f92f44f-7e09-4252-991e-2db268fce266\"}]},\"type\":\"RecordBlkView.InputSignals\",\"uuid\":\"66a969ea-26f5-4669-a233-38bd8f733c60\"}],\"packageUris\":[\"http://schema.mathworks.com/mf0/streamout_blocks/R2020a\"],\"version\":\"1.0\"}"  VisualizationBindings="{\"xyplotplugin\":{\"info\":[{\"series\":[{\"bindingParametersList\":[{\"parameter\":\"X-Axis\",\"signalID\":898,\"signalName\":\"n\"},{\"parameter\":\"Y-Axis\",\"signalID\":901,\"signalName\":\"Mh\"}],\"seriesID\":35191}],\"subplotID\":1}]}}"  CompatibilityTag=XY
  d_i_1alpha : Subsystem
  d_i_1beta : Subsystem
  d_psi_2alpha : Subsystem
  d_psi_2beta : Subsystem
  i2 : Subsystem
  Omega : Outport
  "Measured Motor Current Ia, Ib, Ic" : Outport  Port=2
  Mhnaci : Outport  Port=3
  wires:
  "Voltage Input Ua, Ub, Uc"/1 -> [voltage_motor_input]
  [Omega] -> Omega/1
  [measured_motor_current] -> "Measured Motor Current Ia, Ib, Ic"/1
  [psi_m_alpha] -> Module of Vector1/1(In1)  "psi_m_alpha"
  [slip] -> Scope14/1, To Workspace11/1  "slip"
  Module of Vector2/1(Out1) -> Scope12/1, To Workspace10/1  "psi_m_alpha_beta_module"
  [i_1beta] -> Module of Vector/2(In2)  "i_1_beta"
  [psi_m_alpha] -> Scope4/1, To Workspace6/1  "psi_m_alpha"
  [i_1alpha] -> Mux8/1, Scope2/1, To Workspace4/1  "I_1_alpha"
  From65/1 -> XY Graph/1  "n"
  From67/1 -> XY Graph1/2  "Mh"
  [Mh] -> Scope13/1  "Mh"
  Module of Vector/1(Out1) -> To Workspace14/1, Scope15/1  "i_alpha_beta_module"
  [M_static] -> Scope13/2, To Workspace12/1  "Mh_static"
  [slip] -> Scope9/1  "slip"
  [u_1beta_motor] -> Scope18/2  "u_1beta_motor"
  [Mh] -> Scope7/1, To Workspace9/1  "Mh"
  [u_1alpha_motor] -> Scope18/1  "u_1alpha_motor"
  [psi_m_beta] -> Module of Vector1/2(In2)  "psi_m_beta"
  Module of Vector1/1(Out1) -> Scope6/1, To Workspace8/1  "psi_m_alpha_beta_module"
  [i_1alpha] -> Module of Vector/1(In1)  "I_1_alpha"
  [psi_2beta] -> Module of Vector2/2(In2)  "psi_2_beta"
  [i_1beta] -> Scope3/1, Mux8/2, To Workspace5/1  "i_1_beta"
  [n] -> To Workspace13/1, Scope8/1  "n"
  [psi_m_beta] -> Scope5/1, To Workspace7/1  "psi_m_beta"
  From69/1 -> XY Graph1/1  "n"
  [Omega] -> Scope1/1, To Workspace3/1  "Omega"
  [psi_2alpha] -> Scope10/1, To Workspace15/1  "psi_2_alpha"
  From62/1 -> XY Graph/2  "Mh_static"
  [psi_2alpha] -> Module of Vector2/1(In1)  "psi_2_alpha"
  [psi_2beta] -> To Workspace16/1, Scope11/1  "psi_2_beta"
  Mux8/1 -> Scope20/1
  Demux1/7 -> d_i_1alpha/7(u_1beta)
  [omega] -> Mux4/5
  Constant6/1 -> Divide2/2
  Demux7/2 -> [i_2beta]
  Constant13/1 -> Divide6/2
  Demux2/3 -> d_i_1beta/3(psi_2alpha)
  [K_ClarkeTransform_motor] -> ?
  1-D Lookup Table2/1 -> Manual Switch1/1
  [i_1alpha_beta] -> i2/3(i_1_alpha_beta)
  d_i_1alpha/1(d_i_1alpha) -> Integrator/1
  Constant4/1 -> Manual Switch1/2
  d_i_1beta/1(d_i_1beta) -> Integrator1/1
  Mh/1(Mh) -> [Mh]  "M"
  Divide6/1 -> [n]
  Demux3/5 -> d_psi_2alpha/5(omega)
  Demux1/2 -> d_i_1alpha/2(i_1beta)
  [i_1alpha] -> Mux7/1
  [psi_2alpha] -> Mh/3(phi_2alpha)
  Demux1/6 -> d_i_1alpha/6(u_1alpha)
  Demux5/7 -> d_psi_2beta/7(u_1beta)
  Demux5/1 -> d_psi_2beta/1(i_1alpha)
  i2/1(i_2alpha_beta) -> Demux7/1, [i_2alpha_beta]
  [i_1beta] -> Mux4/2
  Add2/1 -> Divide4/2
  Slip/1(Slip) -> [slip]
  Demux1/1 -> d_i_1alpha/1(i_1alpha)
  Constant5/1 -> Divide1/2
  Demux3/1 -> d_psi_2alpha/1(i_1alpha)
  Mux4/1 -> [FirstStateEquationVariables]
  [FirstStateEquationVariables] -> Demux5/1
  Integrator4/1 -> Divide3/1, [omega]  "omega"
  Manual Switch1/1 -> Manual Switch/1
  Constant10/1 -> Divide3/2
  Demux3/4 -> d_psi_2alpha/4(psi_2beta)
  Demux7/1 -> [i_2alpha]
  Add1/1 -> Divide1/1
  Demux5/5 -> d_psi_2beta/5(omega)
  [Mh] -> Add1/1
  Demux5/4 -> d_psi_2beta/4(psi_2beta)
  d_psi_2beta/1(d_psi_2beta) -> Integrator3/1
  [u_1beta_motor] -> Mux4/7
  Demux8/1 -> [psi_m_alpha]
  [i_1alpha_beta] -> Add2/1
  [i_1alpha] -> Mh/1(i_1alpha)
  Demux1/5 -> d_i_1alpha/5(omega)
  Demux2/6 -> d_i_1beta/6(u_1alpha)
  Demux2/2 -> d_i_1beta/2(i_1beta)
  Mux7/1 -> [i_1alpha_beta]
  [psi_2beta] -> i2/2(psi_2beta)
  Integrator2/1 -> [psi_2alpha]  "psi_2alpha"
  Demux1/4 -> d_i_1alpha/4(psi_2beta)
  Mux6/1 -> [psi_2_alpha_beta]
  [psi_2beta] -> Mh/4(phi_2beta)
  Constant12/1 -> Divide5/2
  1-D Lookup Table/1 -> Manual Switch/2
  Demux6/2 -> Mux/2, [u_1beta_motor]
  Demux3/3 -> d_psi_2alpha/3(psi_2alpha)
  [psi_2beta] -> Mux4/4
  Demux2/4 -> d_i_1beta/4(psi_2beta)
  [i_1beta] -> Mh/2(i_1beta)
  Divide1/1 -> Divide2/1
  Demux5/6 -> d_psi_2beta/6(u_1alpha)
  Demux2/1 -> d_i_1beta/1(i_1alpha)
  [i_2alpha_beta] -> Add2/2
  d_psi_2alpha/1(d_psi_2alpha) -> Integrator2/1
  Manual Switch/1 -> ?
  Divide2/1 -> Integrator4/1  "d_omega"
  [psi_2beta] -> Mux6/2
  Demux5/2 -> d_psi_2beta/2(i_1beta)
  Demux6/1 -> [u_1alpha_motor], Mux/1
  Divide3/1 -> Divide5/1, [Omega]  "d_omega"
  Integrator1/1 -> [i_1beta]  "i_1beta"
  Integrator3/1 -> [psi_2beta]  "psi_2beta"
  [i_1beta] -> Mux7/2
  Constant11/1 -> Divide4/1
  Demux2/5 -> d_i_1beta/5(omega)
  Demux8/2 -> [psi_m_beta]
  Demux3/6 -> d_psi_2alpha/6(u_1alpha)
  [FirstStateEquationVariables] -> Demux1/1
  Integrator/1 -> [i_1alpha]  "i_1alpha"
  [u_1alpha_motor] -> Mux4/6
  [FirstStateEquationVariables] -> Demux3/1
  [psi_2alpha] -> Mux4/3
  [psi_2alpha] -> i2/1(psi_2alpha)
  Divide5/1 -> Divide6/1  "d_omega"
  Demux2/7 -> d_i_1beta/7(u_1beta)
  Demux3/7 -> d_psi_2alpha/7(u_1beta)
  [slip] -> Mh Static/1(Slip)
  Demux3/2 -> d_psi_2alpha/2(i_1beta)
  Demux1/3 -> d_i_1alpha/3(psi_2alpha)
  [voltage_motor_input] -> Clarke Transform/1
  [FirstStateEquationVariables] -> Demux2/1
  Mh Static/1(Mh Static) -> [M_static]
  [psi_2alpha] -> Mux6/1
  [i_1alpha] -> Mux4/1
  [omega] -> Slip/1(omega)  "omega"
  Clock/1 -> 1-D Lookup Table2/1, 1-D Lookup Table/1
  Demux5/3 -> d_psi_2beta/3(psi_2alpha)
  Divide4/1 -> Demux8/1, [psi_m_alpha_beta]
  Clarke Transform/1 -> Demux6/1
  Mux/1 -> [u1_in_alpha_beta_motor]
  [i_1alpha] -> Mux1/1
  [i_1beta] -> Mux1/2
  Constant/1 -> Mux1/3
  Mux1/1 -> Inverse Clarke Transform/1
  Inverse Clarke Transform/1 -> [measured_motor_current]
  Mz/1 -> [Mz]
  [Mz] -> Add1/2
  [Mh] -> Mhnaci/1

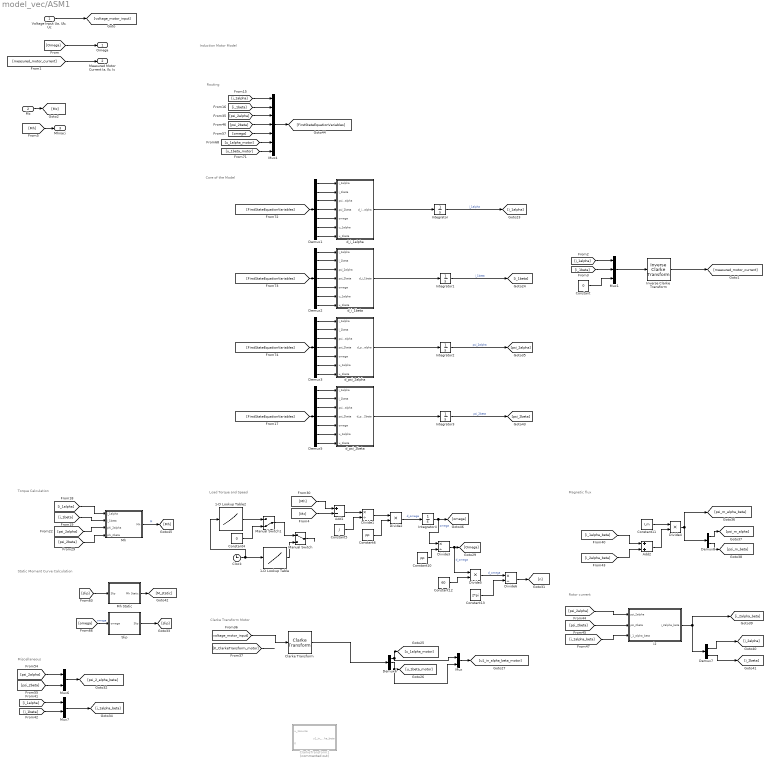
== system model_vec/ASM1 ==
  note: Core of the Model
  note: Torque Calculation
  note: Load Torque and Speed
  note: Miscellaneous
  note: Routing
  note: Static Moment Curve Calculation
  note: Magnetic flux
  note: Rotor current
  note: Induction Motor Model
  note: Clarke Transform Motor
  "Voltage Input Ua, Ub, Uc" : Inport
  Mz : Inport  Port=2
  1-D Lookup Table : Lookup_n-D  NumberOfTableDimensions=1  BreakpointsForDimension1=[0;1.00001;1.001;10]  Table=[0;0;25;25]  InternalRulePriority=Speed  RndMeth=Simplest
  1-D Lookup Table2 : Lookup_n-D  NumberOfTableDimensions=1  BreakpointsForDimension1=[1;2;10]  Table=[0;0;78.48]  InternalRulePriority=Speed  RndMeth=Simplest
  Add1 : Sum  Inputs=+-
  Add2 : Sum
  Clarke Transform : eeTransforms/Clarke Transform  PowerInvariant=off
      settings: LibrarySourceBlock=|
      | ee_sl_lib/Mathematical
      | Transforms/Clarke Transform
  ClarkeTransform1 : Subsystem  Commented=on
  Clock : Clock
  Constant : Constant  Value=0
  Constant10 : Constant  Value=pp
  Constant11 : Constant  Value=Lm
  Constant12 : Constant  Value=60
  Constant13 : Constant  Value=2*pi
  Constant4 : Constant  Value=0
  Constant5 : Constant  Value=J
  Constant6 : Constant  Value=pp
  Demux{1..3,5} (4 alike) : Demux  Outputs=7
  Demux6 : Demux  Outputs=3
  Demux7 : Demux  Outputs=2
  Demux8 : Demux  Outputs=2
  Divide1 : Product  Inputs=*/
  Divide2 : Product  Inputs=**
  Divide3 : Product  Inputs=*/
  Divide4 : Product  Inputs=**
  Divide5 : Product  Inputs=**
  Divide6 : Product  Inputs=*/
  Integrator{,1..4} (5 alike) : Integrator
  Inverse Clarke Transform : eeTransforms/Inverse Clarke Transform  PowerInvariant=off
      settings: LibrarySourceBlock=|
      | ee_sl_lib/Mathematical
      | Transforms/Inverse
      | Clarke Transform
  Manual Switch : ManualSwitch
  Manual Switch1 : ManualSwitch  CurrentSetting=0
  Mh : Subsystem
  Mh Static : Subsystem
  Mux : Mux  Inputs=2
  Mux1 : Mux  Inputs=3
  Mux4 : Mux  Inputs=7
  Mux6 : Mux  Inputs=2
  Mux7 : Mux  Inputs=2
  Slip : Subsystem
  d_i_1alpha : Subsystem
  d_i_1beta : Subsystem
  d_psi_2alpha : Subsystem
  d_psi_2beta : Subsystem
  i2 : Subsystem
  Omega : Outport
  "Measured Motor Current Ia, Ib, Ic" : Outport  Port=2
  Mhnaci : Outport  Port=3
  wires:
  Inverse Clarke Transform/1 -> [measured_motor_current]
  Mux1/1 -> Inverse Clarke Transform/1
  Constant/1 -> Mux1/3
  [i_1beta] -> Mux1/2
  [i_1alpha] -> Mux1/1
  Mux/1 -> [u1_in_alpha_beta_motor]
  Clarke Transform/1 -> Demux6/1
  Divide4/1 -> [psi_m_alpha_beta], Demux8/1
  Demux5/3 -> d_psi_2beta/3(psi_2alpha)
  Clock/1 -> 1-D Lookup Table/1, 1-D Lookup Table2/1
  [omega] -> Slip/1(omega)  "omega"
  [i_1alpha] -> Mux4/1
  [psi_2alpha] -> Mux6/1
  Mh Static/1(Mh Static) -> [M_static]
  [FirstStateEquationVariables] -> Demux2/1
  [voltage_motor_input] -> Clarke Transform/1
  Demux1/3 -> d_i_1alpha/3(psi_2alpha)
  Demux3/2 -> d_psi_2alpha/2(i_1beta)
  [slip] -> Mh Static/1(Slip)
  Demux3/7 -> d_psi_2alpha/7(u_1beta)
  Demux2/7 -> d_i_1beta/7(u_1beta)
  Divide5/1 -> Divide6/1  "d_omega"
  [psi_2alpha] -> i2/1(psi_2alpha)
  [psi_2alpha] -> Mux4/3
  [FirstStateEquationVariables] -> Demux3/1
  [u_1alpha_motor] -> Mux4/6
  Integrator/1 -> [i_1alpha]  "i_1alpha"
  [FirstStateEquationVariables] -> Demux1/1
  Demux3/6 -> d_psi_2alpha/6(u_1alpha)
  Demux8/2 -> [psi_m_beta]
  Demux2/5 -> d_i_1beta/5(omega)
  Constant11/1 -> Divide4/1
  [i_1beta] -> Mux7/2
  Integrator3/1 -> [psi_2beta]  "psi_2beta"
  Integrator1/1 -> [i_1beta]  "i_1beta"
  Divide3/1 -> [Omega], Divide5/1  "d_omega"
  Demux6/1 -> Mux/1, [u_1alpha_motor]
  Demux5/2 -> d_psi_2beta/2(i_1beta)
  [psi_2beta] -> Mux6/2
  Divide2/1 -> Integrator4/1  "d_omega"
  Manual Switch/1 -> ?
  d_psi_2alpha/1(d_psi_2alpha) -> Integrator2/1
  [i_2alpha_beta] -> Add2/2
  Demux2/1 -> d_i_1beta/1(i_1alpha)
  Demux5/6 -> d_psi_2beta/6(u_1alpha)
  Divide1/1 -> Divide2/1
  [i_1beta] -> Mh/2(i_1beta)
  Demux2/4 -> d_i_1beta/4(psi_2beta)
  [psi_2beta] -> Mux4/4
  Demux3/3 -> d_psi_2alpha/3(psi_2alpha)
  Demux6/2 -> [u_1beta_motor], Mux/2
  1-D Lookup Table/1 -> Manual Switch/2
  Constant12/1 -> Divide5/2
  [psi_2beta] -> Mh/4(phi_2beta)
  Mux6/1 -> [psi_2_alpha_beta]
  Demux1/4 -> d_i_1alpha/4(psi_2beta)
  Integrator2/1 -> [psi_2alpha]  "psi_2alpha"
  [psi_2beta] -> i2/2(psi_2beta)
  Mux7/1 -> [i_1alpha_beta]
  Demux2/2 -> d_i_1beta/2(i_1beta)
  Demux2/6 -> d_i_1beta/6(u_1alpha)
  Demux1/5 -> d_i_1alpha/5(omega)
  [i_1alpha] -> Mh/1(i_1alpha)
  [i_1alpha_beta] -> Add2/1
  Demux8/1 -> [psi_m_alpha]
  [u_1beta_motor] -> Mux4/7
  d_psi_2beta/1(d_psi_2beta) -> Integrator3/1
  Demux5/4 -> d_psi_2beta/4(psi_2beta)
  [Mh] -> Add1/1
  Demux5/5 -> d_psi_2beta/5(omega)
  Add1/1 -> Divide1/1
  Demux7/1 -> [i_2alpha]
  Demux3/4 -> d_psi_2alpha/4(psi_2beta)
  Constant10/1 -> Divide3/2
  Manual Switch1/1 -> Manual Switch/1
  Integrator4/1 -> [omega], Divide3/1  "omega"
  [FirstStateEquationVariables] -> Demux5/1
  Mux4/1 -> [FirstStateEquationVariables]
  Demux3/1 -> d_psi_2alpha/1(i_1alpha)
  Constant5/1 -> Divide1/2
  Demux1/1 -> d_i_1alpha/1(i_1alpha)
  Slip/1(Slip) -> [slip]
  Add2/1 -> Divide4/2
  [i_1beta] -> Mux4/2
  i2/1(i_2alpha_beta) -> [i_2alpha_beta], Demux7/1
  Demux5/1 -> d_psi_2beta/1(i_1alpha)
  Demux5/7 -> d_psi_2beta/7(u_1beta)
  Demux1/6 -> d_i_1alpha/6(u_1alpha)
  [psi_2alpha] -> Mh/3(phi_2alpha)
  [i_1alpha] -> Mux7/1
  Demux1/2 -> d_i_1alpha/2(i_1beta)
  Demux3/5 -> d_psi_2alpha/5(omega)
  Divide6/1 -> [n]
  Mh/1(Mh) -> [Mh]  "M"
  d_i_1beta/1(d_i_1beta) -> Integrator1/1
  Constant4/1 -> Manual Switch1/2
  d_i_1alpha/1(d_i_1alpha) -> Integrator/1
  [i_1alpha_beta] -> i2/3(i_1_alpha_beta)
  1-D Lookup Table2/1 -> Manual Switch1/1
  [K_ClarkeTransform_motor] -> ?
  Demux2/3 -> d_i_1beta/3(psi_2alpha)
  Constant13/1 -> Divide6/2
  Demux7/2 -> [i_2beta]
  Constant6/1 -> Divide2/2
  [omega] -> Mux4/5
  Demux1/7 -> d_i_1alpha/7(u_1beta)
  [measured_motor_current] -> "Measured Motor Current Ia, Ib, Ic"/1
  [Omega] -> Omega/1
  "Voltage Input Ua, Ub, Uc"/1 -> [voltage_motor_input]
  Mz/1 -> [Mz]
  [Mh] -> Mhnaci/1
  [Mz] -> Add1/2
